simulink model "schema"  (R2021a)
settings: Solver=ode1  StartTime=0.0  StopTime=inf  FixedStep=0.01  RelTol=1e-3
values from neighbouring files (symbols this model uses):
  FKR_data_len = ceil(((FKR_resolution+1)*FKR_encoder_count)/8)    [fkReaderSetup.m]
libraries: instrumentseriallib x3
settings Model: Creator=Petr  LastModifiedBy=Petr
settings RTWCC: GenerateReport=on  LaunchReport=on

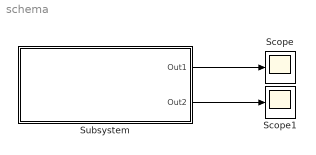
== system schema ==
  Scope : Scope
  Scope1 : Scope
  Subsystem : Subsystem
  wires:
  Subsystem/2(Out2) -> Scope1/1
  Subsystem/1(Out1) -> Scope/1

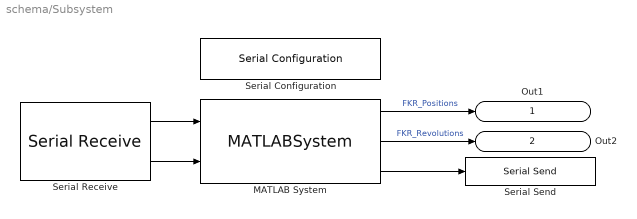
== system schema/Subsystem ==
  MATLAB System : MATLABSystem  System=fkReader  EncoderVector=FKR_encoder_vector  Resolution=FKR_resolution  RevBitDepth=FKR_revolution_bit_depth  DataLen=FKR_data_len  ConfigMessage=FKR_config_message  SimulateUsing=Code generation
      mask Type: fkReader
      mask Display:
      | disp('fkReader');
      | port_label('input',1,'Serial Data In');
      | port_label('input',2,'Serial Status');
      | port_label('output',1,'Positions');
      | port_label('output',2,'Revolutions');
      | port_label('output',3,'SerialOut');
  Serial Configuration : instrumentseriallib/Serial Configuration  Priority=-200000  Port=COM4  ComPort=COM4  BaudRate=FKR_baudrate  DataBits=8  Parity=none  StopBits=1  ByteOrder=little-endian  FlowControl=none  Timeout=10  SimulateUsing=Interpreted execution  BlockInModel=on
  Serial Receive : instrumentseriallib/Serial Receive  Priority=1  Port=COM4  ComPort=COM4  DataType=uint8  SaveDataType=uint8  ToggleHeader=on  Header=FKR_header  ToggleTerminator=off  Terminator=<none>  CustomTerminator=[]  ToggleDataSize=on  DataSize=[1, (FKR_data_len)]  EnableBlockingMode=off  ActionDataUnavailable=Output last received value  ActionWhenDataUnavailable=Output last received value  CustomValue=0  SampleTime=-1  SimulateUsing=Interpreted execution  BlockInModel=on
  Serial Send : instrumentseriallib/Serial Send  Priority=1  Port=COM4  ComPort=COM4  Header=[]  Terminator=<none>  CustomTerminator=[]  EnableBlockingMode=off  SimulateUsing=Interpreted execution  BlockInModel=on
  Out1 : Outport
  Out2 : Outport  Port=2
  wires:
  MATLAB System/2 -> Out2/1  "FKR_Revolutions"
  MATLAB System/3 -> Serial Send/1
  MATLAB System/1 -> Out1/1  "FKR_Positions"
  Serial Receive/1 -> MATLAB System/1
  Serial Receive/2 -> MATLAB System/2
